simulink model "SingleTrack"  (Simulink 7.5)
settings: Solver=ode45  SolverMode=SingleTasking  StartTime=0.0  StopTime=inf  FixedStep=0.001  RelTol=1e-3
PreLoadFcn:
  | SingleTrack_params
undefined symbols (not defined in the file): Car_Bdy1_mass, Car_Steering_i, Car_Whl_Radius, Car_WhlBaseF, Car_WhlBaseR, mEngineMax, PT_DL_iDiff, PT_GearBox_iForwardGears
libraries: CarMaker4SL x8, simulink x6
(part 2 of 4)

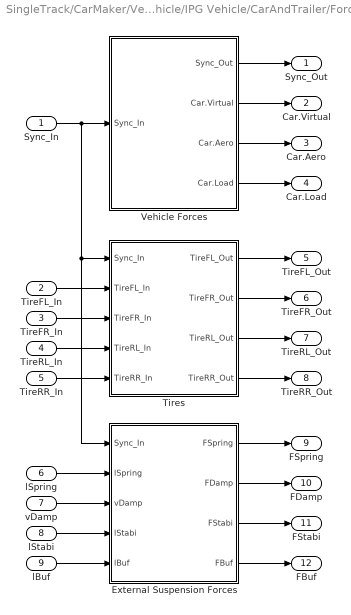
== system SingleTrack/CarMaker/Vehicle/IPG Vehicle/CarAndTrailer/Forces ==
  Sync_In : Inport  OutDataType=sfix(16)  OutScaling=2^0
  TireFL_In : Inport  Port=2  OutDataType=sfix(16)  OutScaling=2^0
  TireFR_In : Inport  Port=3  OutDataType=sfix(16)  OutScaling=2^0
  TireRL_In : Inport  Port=4  OutDataType=sfix(16)  OutScaling=2^0
  TireRR_In : Inport  Port=5  OutDataType=sfix(16)  OutScaling=2^0
  lSpring : Inport  Port=6  OutDataType=sfix(16)  OutScaling=2^0
  vDamp : Inport  Port=7  OutDataType=sfix(16)  OutScaling=2^0
  lStabi : Inport  Port=8  OutDataType=sfix(16)  OutScaling=2^0
  lBuf : Inport  Port=9  OutDataType=sfix(16)  OutScaling=2^0
  External Suspension Forces : Subsystem
  Tires : Subsystem
  Vehicle Forces : Subsystem
  Sync_Out : Outport  OutDataType=sfix(16)  OutScaling=2^0
  Car.Virtual : Outport  Port=2  OutDataType=sfix(16)  OutScaling=2^0
  Car.Aero : Outport  Port=3  OutDataType=sfix(16)  OutScaling=2^0
  Car.Load : Outport  Port=4  OutDataType=sfix(16)  OutScaling=2^0
  TireFL_Out : Outport  Port=5  OutDataType=sfix(16)  OutScaling=2^0
  TireFR_Out : Outport  Port=6  OutDataType=sfix(16)  OutScaling=2^0
  TireRL_Out : Outport  Port=7  OutDataType=sfix(16)  OutScaling=2^0
  TireRR_Out : Outport  Port=8  OutDataType=sfix(16)  OutScaling=2^0
  FSpring : Outport  Port=9  OutDataType=sfix(16)  OutScaling=2^0
  FDamp : Outport  Port=10  OutDataType=sfix(16)  OutScaling=2^0
  FStabi : Outport  Port=11  OutDataType=sfix(16)  OutScaling=2^0
  FBuf : Outport  Port=12  OutDataType=sfix(16)  OutScaling=2^0
  wires:
  External Suspension Forces/1(FSpring) -> FSpring/1
  External Suspension Forces/3(FStabi) -> FStabi/1
  lStabi/1 -> External Suspension Forces/4(lStabi)
  vDamp/1 -> External Suspension Forces/3(vDamp)
  External Suspension Forces/2(FDamp) -> FDamp/1
  lSpring/1 -> External Suspension Forces/2(lSpring)
  Vehicle Forces/4(Car.Load) -> Car.Load/1
  Vehicle Forces/3(Car.Aero) -> Car.Aero/1
  Vehicle Forces/2(Car.Virtual) -> Car.Virtual/1
  TireFL_In/1 -> Tires/2(TireFL_In)
  Vehicle Forces/1(Sync_Out) -> Sync_Out/1
  Sync_In/1 -> Vehicle Forces/1(Sync_In), External Suspension Forces/1(Sync_In), Tires/1(Sync_In)
  TireFR_In/1 -> Tires/3(TireFR_In)
  TireRL_In/1 -> Tires/4(TireRL_In)
  TireRR_In/1 -> Tires/5(TireRR_In)
  Tires/1(TireFL_Out) -> TireFL_Out/1
  Tires/2(TireFR_Out) -> TireFR_Out/1
  Tires/3(TireRL_Out) -> TireRL_Out/1
  Tires/4(TireRR_Out) -> TireRR_Out/1
  lBuf/1 -> External Suspension Forces/5(lBuf)
  External Suspension Forces/4(FBuf) -> FBuf/1

== system SingleTrack/CarMaker/Vehicle/IPG Vehicle/CarAndTrailer/Kinematics ==
  Sync_In : Inport  OutDataType=sfix(16)  OutScaling=2^0
  Steer.IF : Inport  Port=2  OutDataType=sfix(16)  OutScaling=2^0
  Kinematics : S-Function  FunctionName=CM_Sfun  Parameters='Kinematics'  EnableBusSupport=off
  Sync_Out : Outport  OutDataType=sfix(16)  OutScaling=2^0
  TireFL_In : Outport  Port=2  OutDataType=sfix(16)  OutScaling=2^0
  TireFR_In : Outport  Port=3  OutDataType=sfix(16)  OutScaling=2^0
  TireRL_In : Outport  Port=4  OutDataType=sfix(16)  OutScaling=2^0
  TireRR_In : Outport  Port=5  OutDataType=sfix(16)  OutScaling=2^0
  lSpring : Outport  Port=6  OutDataType=sfix(16)  OutScaling=2^0
  vDamp : Outport  Port=7  OutDataType=sfix(16)  OutScaling=2^0
  lStabi : Outport  Port=8  OutDataType=sfix(16)  OutScaling=2^0
  lBuf : Outport  Port=9  OutDataType=sfix(16)  OutScaling=2^0
  wires:
  Steer.IF/1 -> Kinematics/2
  Kinematics/1 -> Sync_Out/1
  Sync_In/1 -> Kinematics/1
  Kinematics/7 -> vDamp/1
  Kinematics/6 -> lSpring/1
  Kinematics/5 -> TireRR_In/1
  Kinematics/4 -> TireRL_In/1
  Kinematics/3 -> TireFR_In/1
  Kinematics/2 -> TireFL_In/1
  Kinematics/8 -> lStabi/1
  Kinematics/9 -> lBuf/1

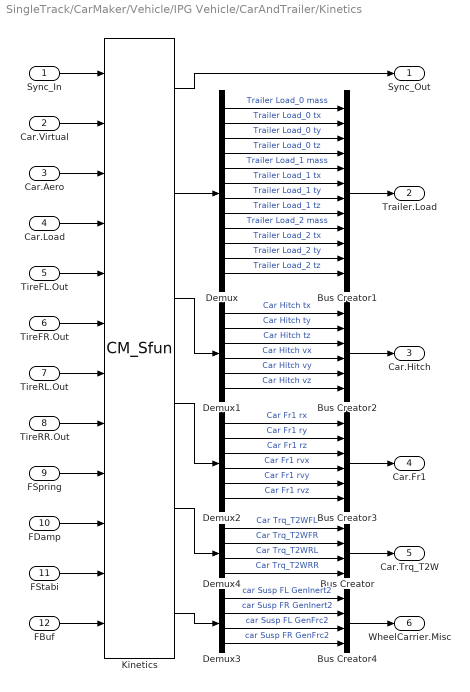
== system SingleTrack/CarMaker/Vehicle/IPG Vehicle/CarAndTrailer/Kinetics ==
  Sync_In : Inport  OutDataType=sfix(16)  OutScaling=2^0
  Car.Virtual : Inport  Port=2  OutDataType=sfix(16)  OutScaling=2^0
  Car.Aero : Inport  Port=3  OutDataType=sfix(16)  OutScaling=2^0
  Car.Load : Inport  Port=4  OutDataType=sfix(16)  OutScaling=2^0
  TireFL.Out : Inport  Port=5  OutDataType=sfix(16)  OutScaling=2^0
  TireFR.Out : Inport  Port=6  OutDataType=sfix(16)  OutScaling=2^0
  TireRL.Out : Inport  Port=7  OutDataType=sfix(16)  OutScaling=2^0
  TireRR.Out : Inport  Port=8  OutDataType=sfix(16)  OutScaling=2^0
  FSpring : Inport  Port=9  OutDataType=sfix(16)  OutScaling=2^0
  FDamp : Inport  Port=10  OutDataType=sfix(16)  OutScaling=2^0
  FStabi : Inport  Port=11  OutDataType=sfix(16)  OutScaling=2^0
  FBuf : Inport  Port=12  OutDataType=sfix(16)  OutScaling=2^0
  Bus Creator : BusCreator
  Bus Creator1 : BusCreator  Inputs=12
  Bus Creator2 : BusCreator  Inputs=6
  Bus Creator3 : BusCreator  Inputs=6
  Bus Creator4 : BusCreator
  Demux : Demux  Outputs=12
  Demux1 : Demux  Outputs=6
  Demux2 : Demux  Outputs=6
  Demux3 : Demux
  Demux4 : Demux
  Kinetics : S-Function  FunctionName=CM_Sfun  Parameters='Kinetics'  EnableBusSupport=off
  Sync_Out : Outport  OutDataType=sfix(16)  OutScaling=2^0
  Trailer.Load : Outport  Port=2  OutDataType=sfix(16)  OutScaling=2^0
  Car.Hitch : Outport  Port=3  OutDataType=sfix(16)  OutScaling=2^0
  Car.Fr1 : Outport  Port=4  OutDataType=sfix(16)  OutScaling=2^0
  Car.Trq_T2W : Outport  Port=5  OutDataType=sfix(16)  OutScaling=2^0
  WheelCarrier.Misc : Outport  Port=6  OutDataType=sfix(16)  OutScaling=2^0
  wires:
  Kinetics/5 -> Demux4/1
  Kinetics/6 -> Demux3/1
  FStabi/1 -> Kinetics/11
  FDamp/1 -> Kinetics/10
  FSpring/1 -> Kinetics/9
  TireRR.Out/1 -> Kinetics/8
  TireRL.Out/1 -> Kinetics/7
  TireFR.Out/1 -> Kinetics/6
  TireFL.Out/1 -> Kinetics/5
  Demux4/1 -> Bus Creator/1  "Car Trq_T2WFL"
  Demux4/2 -> Bus Creator/2  "Car Trq_T2WFR"
  Demux4/3 -> Bus Creator/3  "Car Trq_T2WRL"
  Demux4/4 -> Bus Creator/4  "Car Trq_T2WRR"
  Bus Creator/1 -> Car.Trq_T2W/1
  Bus Creator4/1 -> WheelCarrier.Misc/1
  Demux3/4 -> Bus Creator4/4  "car Susp FR GenFrc2"
  Demux3/3 -> Bus Creator4/3  "car Susp FL GenFrc2"
  Demux3/2 -> Bus Creator4/2  "car Susp FR GenInert2"
  Demux3/1 -> Bus Creator4/1  "car Susp FL GenInert2"
  Car.Load/1 -> Kinetics/4
  Kinetics/4 -> Demux2/1
  Bus Creator3/1 -> Car.Fr1/1
  Demux2/6 -> Bus Creator3/6  "Car Fr1 rvz"
  Demux2/5 -> Bus Creator3/5  "Car Fr1 rvy"
  Demux2/4 -> Bus Creator3/4  "Car Fr1 rvx"
  Demux2/3 -> Bus Creator3/3  "Car Fr1 rz"
  Demux2/2 -> Bus Creator3/2  "Car Fr1 ry"
  Demux2/1 -> Bus Creator3/1  "Car Fr1 rx"
  Bus Creator2/1 -> Car.Hitch/1
  Kinetics/3 -> Demux1/1
  Demux1/6 -> Bus Creator2/6  "Car Hitch vz"
  Demux1/5 -> Bus Creator2/5  "Car Hitch vy"
  Demux1/4 -> Bus Creator2/4  "Car Hitch vx"
  Demux1/3 -> Bus Creator2/3  "Car Hitch tz"
  Demux1/2 -> Bus Creator2/2  "Car Hitch ty"
  Demux1/1 -> Bus Creator2/1  "Car Hitch tx"
  Demux/12 -> Bus Creator1/12  "Trailer Load_2 tz"
  Demux/11 -> Bus Creator1/11  "Trailer Load_2 ty"
  Demux/10 -> Bus Creator1/10  "Trailer Load_2 tx"
  Demux/9 -> Bus Creator1/9  "Trailer Load_2 mass"
  Demux/8 -> Bus Creator1/8  "Trailer Load_1 tz"
  Demux/7 -> Bus Creator1/7  "Trailer Load_1 ty"
  Demux/6 -> Bus Creator1/6  "Trailer Load_1 tx"
  Demux/5 -> Bus Creator1/5  "Trailer Load_1 mass"
  Kinetics/2 -> Demux/1
  Demux/4 -> Bus Creator1/4  "Trailer Load_0 tz"
  Demux/3 -> Bus Creator1/3  "Trailer Load_0 ty"
  Demux/2 -> Bus Creator1/2  "Trailer Load_0 tx"
  Demux/1 -> Bus Creator1/1  "Trailer Load_0 mass"
  Bus Creator1/1 -> Trailer.Load/1
  Car.Virtual/1 -> Kinetics/2
  Car.Aero/1 -> Kinetics/3
  Kinetics/1 -> Sync_Out/1
  Sync_In/1 -> Kinetics/1
  FBuf/1 -> Kinetics/12

== system SingleTrack/CarMaker/Vehicle/IPG Vehicle/CarAndTrailer/Steering ==
  note: When replacing the entire steering system,
      | be sure to add '-disablesteering' to the command line arguments
      | in the CarMaker Model Configuration block.
  Sync_In : Inport  OutDataType=sfix(16)  OutScaling=2^0
  VhclCtrl.Steering : Inport  Port=2  OutDataType=sfix(16)  OutScaling=2^0
  Bus Creator1 : BusCreator  Inputs=16
  Bus Creator2 : BusCreator
  Demux : Demux  Outputs=20
  Steering : S-Function  FunctionName=CM_Sfun  Parameters='Steering'  EnableBusSupport=off
  Terminator : Terminator
  Sync_Out : Outport  OutDataType=sfix(16)  OutScaling=2^0
  Steer.IF : Outport  Port=2  OutDataType=sfix(16)  OutScaling=2^0
  wires:
  Demux/5 -> Bus Creator1/5  "Steering IF TrqStatic"
  Demux/4 -> Bus Creator1/4  "Steering IF Trq"
  Demux/3 -> Bus Creator1/3  "Steering IF AngAcc"
  Demux/2 -> Bus Creator1/2  "Steering IF AngVel"
  Demux/1 -> Bus Creator1/1  "Steering IF Ang"
  Sync_In/1 -> Steering/1
  Steering/1 -> Sync_Out/1
  VhclCtrl.Steering/1 -> Steering/2
  Demux/15 -> Bus Creator1/15  "Steering IF R qpp"
  Demux/14 -> Bus Creator1/14  "Steering IF R qp"
  Demux/13 -> Bus Creator1/13  "Steering IF R q"
  Demux/12 -> Bus Creator1/12  "Steering IF L iSteer2q"
  Demux/11 -> Bus Creator1/11  "Steering IF L qpp"
  Demux/10 -> Bus Creator1/10  "Steering IF L qp"
  Demux/9 -> Bus Creator1/9  "Steering IF L q"
  Demux/16 -> Bus Creator1/16  "Steering IF R iSteer2q"
  Bus Creator2/1 -> Terminator/1  "Steer IF (in)"
  Demux/19 -> Bus Creator2/3  "Steering IF R Frc"
  Demux/18 -> Bus Creator2/2  "Steering IF L Inert"
  Demux/17 -> Bus Creator2/1  "Steering IF L Frc"
  Demux/20 -> Bus Creator2/4  "Steering IF R Inert"
  Demux/6 -> Bus Creator1/6  "Steering IF AssistFrc"
  Demux/7 -> Bus Creator1/7  "Steering IF AssistTrqCol"
  Demux/8 -> Bus Creator1/8  "Steering IF AssistTrqPin"
  Steering/2 -> Demux/1
  Bus Creator1/1 -> Steer.IF/1

== system SingleTrack/CarMaker/Vehicle/IPG Vehicle/CarAndTrailer/Trailer ==
  Sync_In : Inport  OutDataType=sfix(16)  OutScaling=2^0
  Trailer.Load : Inport  Port=2  OutDataType=sfix(16)  OutScaling=2^0
  Car.Hitch : Inport  Port=3  OutDataType=sfix(16)  OutScaling=2^0
  Car.Fr1 : Inport  Port=4  OutDataType=sfix(16)  OutScaling=2^0
  Car.Trq_T2W : Inport  Port=5  OutDataType=sfix(16)  OutScaling=2^0
  WheelCarrier.Misc : Inport  Port=6  OutDataType=sfix(16)  OutScaling=2^0
  CreateBus Car.Hitch.FrcTrq : Subsystem
  CreateBus Vhcl.Motion : Subsystem
  CreateBus Vhcl.PoI : Subsystem
  CreateBus Vhcl.Steering : Subsystem
  CreateBus Vhcl.Wheel.FL : Subsystem
  CreateBus Vhcl.Wheel.FR : Subsystem
  CreateBus Vhcl.Wheel.RL : Subsystem
  CreateBus Vhcl.Wheel.RR : Subsystem
  Trailer : S-Function  FunctionName=CM_Sfun  Parameters='Trailer'  EnableBusSupport=off
  Sync_Out : Outport  OutDataType=sfix(16)  OutScaling=2^0
  Vhcl.Steering : Outport  Port=2  OutDataType=sfix(16)  OutScaling=2^0
  Vhcl.Motion : Outport  Port=3  OutDataType=sfix(16)  OutScaling=2^0
  Vhcl.PoI : Outport  Port=4  OutDataType=sfix(16)  OutScaling=2^0
  Vhcl.Wheel.FL : Outport  Port=5  OutDataType=sfix(16)  OutScaling=2^0
  Vhcl.Wheel.FR : Outport  Port=6  OutDataType=sfix(16)  OutScaling=2^0
  Vhcl.Wheel.RL : Outport  Port=7  OutDataType=sfix(16)  OutScaling=2^0
  Vhcl.Wheel.RR : Outport  Port=8  OutDataType=sfix(16)  OutScaling=2^0
  Car.Hitch.FrcTrq : Outport  Port=9  OutDataType=sfix(16)  OutScaling=2^0
  wires:
  Sync_In/1 -> Trailer/1
  Trailer/1 -> Sync_Out/1
  Trailer.Load/1 -> Trailer/2
  Car.Hitch/1 -> Trailer/3
  Car.Fr1/1 -> Trailer/4
  CreateBus Car.Hitch.FrcTrq/1(Car.Hitch.FrcTrq) -> Car.Hitch.FrcTrq/1
  WheelCarrier.Misc/1 -> Trailer/6
  Car.Trq_T2W/1 -> Trailer/5
  CreateBus Vhcl.Motion/1(Out1) -> Vhcl.Motion/1
  CreateBus Vhcl.PoI/1(Out1) -> Vhcl.PoI/1
  CreateBus Vhcl.Wheel.FL/1(Out1) -> Vhcl.Wheel.FL/1  "Vhcl.Wheel.FL"
  CreateBus Vhcl.Wheel.FR/1(Out1) -> Vhcl.Wheel.FR/1  "Vhcl.Wheel.FR"
  CreateBus Vhcl.Wheel.RL/1(Out1) -> Vhcl.Wheel.RL/1  "Vhcl.Wheel.RL"
  CreateBus Vhcl.Wheel.RR/1(Out1) -> Vhcl.Wheel.RR/1  "Vhcl.Wheel.RR"
  Trailer/8 -> CreateBus Vhcl.Wheel.RR/1(In1)
  Trailer/9 -> CreateBus Car.Hitch.FrcTrq/1(In1)
  Trailer/7 -> CreateBus Vhcl.Wheel.RL/1(In1)
  Trailer/6 -> CreateBus Vhcl.Wheel.FR/1(In1)
  Trailer/5 -> CreateBus Vhcl.Wheel.FL/1(In1)
  Trailer/4 -> CreateBus Vhcl.PoI/1(In1)
  Trailer/3 -> CreateBus Vhcl.Motion/1(In1)
  CreateBus Vhcl.Steering/1(Out1) -> Vhcl.Steering/1
  Trailer/2 -> CreateBus Vhcl.Steering/1(In1)

== system SingleTrack/CarMaker/Vehicle/User Vehicle (CM4SL)/Brake/CreateBus Vhcl.Wheel.PT ==
  In : Inport
  BusCreator : BusCreator  Inputs=16
  Demux : Demux  Outputs=16
  Out : Outport
  wires:
  In/1 -> Demux/1
  BusCreator/1 -> Out/1
  Demux/1 -> BusCreator/1  "Vhcl Wheel FL Trq_Brake"
  Demux/2 -> BusCreator/2  "Vhcl Wheel FL Trq_BrakeReg_trg"
  Demux/3 -> BusCreator/3  "Vhcl Wheel FL Trq_T2W"
  Demux/4 -> BusCreator/4  "Vhcl Wheel FL WhlBearing"
  Demux/5 -> BusCreator/5  "Vhcl Wheel FR Trq_Brake"
  Demux/6 -> BusCreator/6  "Vhcl Wheel FR Trq_BrakeReg_trg"
  Demux/7 -> BusCreator/7  "Vhcl Wheel FR Trq_T2W"
  Demux/8 -> BusCreator/8  "Vhcl Wheel FR WhlBearing"
  Demux/9 -> BusCreator/9  "Vhcl Wheel RL Trq_Brake"
  Demux/10 -> BusCreator/10  "Vhcl Wheel RL Trq_BrakeReg_trg"
  Demux/11 -> BusCreator/11  "Vhcl Wheel RL Trq_T2W"
  Demux/12 -> BusCreator/12  "Vhcl Wheel RL WhlBearing"
  Demux/13 -> BusCreator/13  "Vhcl Wheel RR Trq_Brake"
  Demux/14 -> BusCreator/14  "Vhcl Wheel RR Trq_BrakeReg_trg"
  Demux/15 -> BusCreator/15  "Vhcl Wheel RR Trq_T2W"
  Demux/16 -> BusCreator/16  "Vhcl Wheel RR WhlBearing"

== system SingleTrack/CarMaker/Vehicle/User Vehicle (CM4SL)/CarAndTrailer/CarAndTrailerUpd1 ==
  Sync_In : Inport  OutDataType=sfix(16)  OutScaling=2^0
  Vhcl.Steering : Inport  Port=2  OutDataType=sfix(16)  OutScaling=2^0
  Vhcl.Motion : Inport  Port=3  OutDataType=sfix(16)  OutScaling=2^0
  Vhcl.PoI : Inport  Port=4  OutDataType=sfix(16)  OutScaling=2^0
  Vhcl.Wheel.FL : Inport  Port=5  OutDataType=sfix(16)  OutScaling=2^0
  Vhcl.Wheel.FR : Inport  Port=6  OutDataType=sfix(16)  OutScaling=2^0
  Vhcl.Wheel.RL : Inport  Port=7  OutDataType=sfix(16)  OutScaling=2^0
  Vhcl.Wheel.RR : Inport  Port=8  OutDataType=sfix(16)  OutScaling=2^0
  Car.Hitch.FrcTrq : Inport  Port=9  OutDataType=sfix(16)  OutScaling=2^0
  Vhcl.Fr1A : Inport  Port=10  OutDataType=sfix(16)  OutScaling=2^0
  CarAndTrailerUpd : S-Function  FunctionName=CM_Sfun  Parameters='CarAndTrUpd'  EnableBusSupport=off
  CreateBus Brake.IF.In : Subsystem
  Sync_Out : Outport  OutDataType=sfix(16)  OutScaling=2^0
  Brake.IF.In : Outport  Port=2  OutDataType=sfix(16)  OutScaling=2^0
  wires:
  Sync_In/1 -> CarAndTrailerUpd/1
  CarAndTrailerUpd/1 -> Sync_Out/1
  CreateBus Brake.IF.In/1(Out) -> Brake.IF.In/1
  CarAndTrailerUpd/2 -> CreateBus Brake.IF.In/1(In)
  Vhcl.Wheel.RL/1 -> CarAndTrailerUpd/7
  Vhcl.Wheel.RR/1 -> CarAndTrailerUpd/8
  Car.Hitch.FrcTrq/1 -> CarAndTrailerUpd/9
  Vhcl.Wheel.FR/1 -> CarAndTrailerUpd/6
  Vhcl.Wheel.FL/1 -> CarAndTrailerUpd/5
  Vhcl.PoI/1 -> CarAndTrailerUpd/4
  Vhcl.Motion/1 -> CarAndTrailerUpd/3
  Vhcl.Steering/1 -> CarAndTrailerUpd/2
  Vhcl.Fr1A/1 -> CarAndTrailerUpd/10  "user vehicle only"

== system SingleTrack/CarMaker/Vehicle/User Vehicle (CM4SL)/CarAndTrailer/CreateBus Car.Hitch.FrcTrq ==
  Bus Creator : BusCreator  Inputs=6
  Constant{1..2,7..10} (6 alike) : Constant  Value=0  OutDataType=sfix(16)  OutScaling=2^0
  Demux7 : Demux  Outputs=6
  Mux1 : Mux  Inputs=6
  Car.Hitch.FrcTrq : Outport  OutDataType=sfix(16)  OutScaling=2^0
  wires:
  Demux7/1 -> Bus Creator/1  "Car Hitch Frc2Car x"
  Demux7/2 -> Bus Creator/2  "Car Hitch Frc2Car y"
  Demux7/3 -> Bus Creator/3  "Car Hitch Frc2Car z"
  Demux7/4 -> Bus Creator/4  "Car Hitch Trq2Car x"
  Demux7/5 -> Bus Creator/5  "Car Hitch Trq2Car y"
  Demux7/6 -> Bus Creator/6  "Car Hitch Trq2Car z"
  Bus Creator/1 -> Car.Hitch.FrcTrq/1
  Mux1/1 -> Demux7/1
  Constant8/1 -> Mux1/2
  Constant9/1 -> Mux1/3
  Constant10/1 -> Mux1/4
  Constant7/1 -> Mux1/1
  Constant2/1 -> Mux1/5
  Constant1/1 -> Mux1/6

== system SingleTrack/CarMaker/Vehicle/User Vehicle (CM4SL)/CarAndTrailer/CreateBus Vhcl.Fr1 ==
  Vhcl.Fr1_In : Inport  OutDataType=sfix(16)  OutScaling=2^0
  BdyFrame2Vhcl.Fr1A : Subsystem
  Ground : Ground
  Ground1 : Ground
  Tr2Fr0 : Subsystem
  a_0 : Subsystem
  t_0 : Subsystem
  v_0 : Subsystem
  Vhcl.Fr1A : Outport  OutDataType=sfix(16)  OutScaling=2^0
  wires:
  BdyFrame2Vhcl.Fr1A/1(Vhcl.Fr1) -> Vhcl.Fr1A/1
  Vhcl.Fr1_In/1 -> a_0/1(Car), v_0/1(Car), t_0/1(Car), Tr2Fr0/1(Car)
  Tr2Fr0/1(Tr2Fr0) -> v_0/2(Tr2Fr0), a_0/2(Tr2Fr0), BdyFrame2Vhcl.Fr1A/6(Tr2Fr0)
  t_0/1(t_0) -> BdyFrame2Vhcl.Fr1A/1(t_0)
  v_0/1(v_0) -> BdyFrame2Vhcl.Fr1A/2(v_0)
  a_0/1(a_0) -> BdyFrame2Vhcl.Fr1A/3(a_0)
  Ground1/1 -> BdyFrame2Vhcl.Fr1A/4(omega_0)
  Ground/1 -> BdyFrame2Vhcl.Fr1A/5(alpha_0)

== system SingleTrack/CarMaker/Vehicle/User Vehicle (CM4SL)/CarAndTrailer/CreateBus Vhcl.Motion ==
  Vhcl_Motion_In : Inport  OutDataType=sfix(16)  OutScaling=2^0
  Bus Creator : BusCreator  Inputs=16
  Bus Selector1 : BusSelector  OutputSignals=Car_vx_1,Car_Dist,Car_sRoad,Road_Fr1_rx,Road_Fr1_ry,Car_Yaw,Car_Yawp,Car_Yawpp
  Constant{1,5,8,11..14} (7 alike) : Constant  Value=0  OutDataType=sfix(16)  OutScaling=2^0
  Demux1 : Demux  Outputs=16
  Mux3 : Mux  Inputs=16
  Vhcl .Motion : Outport  OutDataType=sfix(16)  OutScaling=2^0
  wires:
  Vhcl_Motion_In/1 -> Bus Selector1/1
  Mux3/1 -> Demux1/1
  Bus Creator/1 -> Vhcl .Motion/1
  Demux1/16 -> Bus Creator/16  "Vhcl YawAcc"
  Demux1/15 -> Bus Creator/15  "Vhcl YawRate"
  Demux1/14 -> Bus Creator/14  "Vhcl Yaw"
  Demux1/13 -> Bus Creator/13  "Vhcl PitchAcc"
  Demux1/12 -> Bus Creator/12  "Vhcl PitchVel"
  Demux1/11 -> Bus Creator/11  "Vhcl Pitch"
  Demux1/10 -> Bus Creator/10  "Vhcl RollAcc"
  Demux1/9 -> Bus Creator/9  "Vhcl RollVel"
  Demux1/8 -> Bus Creator/8  "Vhcl Roll"
  Demux1/7 -> Bus Creator/7  "Vhcl Hitch_Pos z"
  Demux1/6 -> Bus Creator/6  "Vhcl Hitch_Pos y"
  Demux1/5 -> Bus Creator/5  "Vhcl Hitch_Pos x"
  Demux1/4 -> Bus Creator/4  "Vhcl sRoadAero"
  Demux1/3 -> Bus Creator/3  "Vhcl sRoad"
  Demux1/2 -> Bus Creator/2  "Vhcl Distance"
  Demux1/1 -> Bus Creator/1  "Vhcl v"
  Bus Selector1/3 -> Mux3/4, Mux3/3  "<Car_sRoad>"
  Bus Selector1/5 -> Mux3/11  "<Road_Fr1_ry>"
  Bus Selector1/4 -> Mux3/8  "<Road_Fr1_rx>"
  Bus Selector1/8 -> Mux3/16  "<Car_Yawpp>"
  Bus Selector1/7 -> Mux3/15  "<Car_Yawp>"
  Bus Selector1/6 -> Mux3/14  "<Car_Yaw>"
  Constant1/1 -> Mux3/13
  Constant14/1 -> Mux3/12
  Constant13/1 -> Mux3/10
  Constant12/1 -> Mux3/9
  Constant11/1 -> Mux3/7
  Constant8/1 -> Mux3/6
  Constant5/1 -> Mux3/5
  Bus Selector1/2 -> Mux3/2  "<Car_Dist>"
  Bus Selector1/1 -> Mux3/1  "<Car_vx_1>"

== system SingleTrack/CarMaker/Vehicle/User Vehicle (CM4SL)/CarAndTrailer/CreateBus Vhcl.PoI ==
  Vhcl_POI_In : Inport  OutDataType=sfix(16)  OutScaling=2^0
  Bus Creator : BusCreator  Inputs=18
  Bus Selector : BusSelector  OutputSignals=Car_x,Car_y,Road_Fr1_z,Car_vx,Car_vy,Car_ax,Car_ay,Car_vx_1,Car_ax_1,Car_ay_1
  Constant{11..13,15..19} (8 alike) : Constant  Value=0  OutDataType=sfix(16)  OutScaling=2^0
  Demux3 : Demux  Outputs=18
  Mux1 : Mux  Inputs=18
  Vhcl.PoI : Outport  OutDataType=sfix(16)  OutScaling=2^0
  wires:
  Demux3/1 -> Bus Creator/1  "Vhcl PoI_Pos x"
  Bus Creator/1 -> Vhcl.PoI/1
  Demux3/2 -> Bus Creator/2  "Vhcl PoI_Pos y"
  Demux3/3 -> Bus Creator/3  "Vhcl PoI_Pos z"
  Demux3/4 -> Bus Creator/4  "Vhcl PoI_Vel x"
  Demux3/5 -> Bus Creator/5  "Vhcl PoI_Vel y"
  Demux3/6 -> Bus Creator/6  "Vhcl PoI_Vel z"
  Demux3/7 -> Bus Creator/7  "Vhcl PoI_Acc x"
  Demux3/8 -> Bus Creator/8  "Vhcl PoI_Acc y"
  Demux3/9 -> Bus Creator/9  "Vhcl PoI_Acc z"
  Demux3/10 -> Bus Creator/10  "Vhcl PoI_Vel_1 x"
  Demux3/11 -> Bus Creator/11  "Vhcl PoI_Vel_1 y"
  Demux3/12 -> Bus Creator/12  "Vhcl PoI_Vel_1 z"
  Demux3/13 -> Bus Creator/13  "Vhcl PoI_Acc_1 x"
  Demux3/14 -> Bus Creator/14  "Vhcl PoI_Acc_1 y"
  Demux3/15 -> Bus Creator/15  "Vhcl PoI_Acc_1 z"
  Demux3/16 -> Bus Creator/16  "Vhcl PoI_GCS Long"
  Demux3/17 -> Bus Creator/17  "Vhcl PoI_GCS Lat"
  Demux3/18 -> Bus Creator/18  "Vhcl PoI_GCS Elev"
  Mux1/1 -> Demux3/1
  Vhcl_POI_In/1 -> Bus Selector/1
  Constant12/1 -> Mux1/16
  Constant13/1 -> Mux1/17
  Constant11/1 -> Mux1/18
  Bus Selector/1 -> Mux1/1  "<Car_x>"
  Bus Selector/2 -> Mux1/2  "<Car_y>"
  Bus Selector/3 -> Mux1/3  "<Road_Fr1_z>"
  Bus Selector/4 -> Mux1/4  "<Car_vx>"
  Bus Selector/5 -> Mux1/5  "<Car_vy>"
  Constant15/1 -> Mux1/6
  Bus Selector/6 -> Mux1/7  "<Car_ax>"
  Constant16/1 -> Mux1/9
  Constant17/1 -> Mux1/11
  Constant18/1 -> Mux1/12
  Bus Selector/9 -> Mux1/13  "<Car_ax_1>"
  Bus Selector/10 -> Mux1/14  "<Car_ay_1>"
  Constant19/1 -> Mux1/15
  Bus Selector/7 -> Mux1/8  "<Car_ay>"
  Bus Selector/8 -> Mux1/10  "<Car_vx_1>"

== system SingleTrack/CarMaker/Vehicle/User Vehicle (CM4SL)/CarAndTrailer/CreateBus Vhcl.Steering ==
  Vhcl_Steering_In : Inport  OutDataType=sfix(16)  OutScaling=2^0
  Bus Creator : BusCreator
  Bus Selector : BusSelector  OutputSignals=VhclCtrl Steering Ang,VhclCtrl Steering AngVel,VhclCtrl Steering AngAcc,VhclCtrl Steering Trq
  Demux : Demux
  Mux1 : Mux
  Vhcl.Steering : Outport  OutDataType=sfix(16)  OutScaling=2^0
  wires:
  Demux/4 -> Bus Creator/4  "Vhcl Steering Trq"
  Demux/2 -> Bus Creator/2  "Vhcl Steering AngVel"
  Demux/3 -> Bus Creator/3  "Vhcl Steering AngAcc"
  Demux/1 -> Bus Creator/1  "Vhcl Steering Ang"
  Bus Creator/1 -> Vhcl.Steering/1
  Vhcl_Steering_In/1 -> Bus Selector/1
  Bus Selector/1 -> Mux1/1  "<VhclCtrl Steering Ang>"
  Bus Selector/2 -> Mux1/2  "<VhclCtrl Steering AngVel>"
  Bus Selector/3 -> Mux1/3  "<VhclCtrl Steering AngAcc>"
  Bus Selector/4 -> Mux1/4  "<VhclCtrl Steering Trq>"
  Mux1/1 -> Demux/1

== system SingleTrack/CarMaker/Vehicle/User Vehicle (CM4SL)/CarAndTrailer/CreateBus Vhcl.Wheel.FL ==
  Vhcl.Wheel.FL_In : Inport  OutDataType=sfix(16)  OutScaling=2^0
  Bus Creator : BusCreator  Inputs=14
  Bus Selector : BusSelector  OutputSignals=Car_Whl_F_rz,Car_Whl_Fz,Car_Whl_F_SideSlip
  Constant{1..6,8..12} (11 alike) : Constant  Value=0  OutDataType=sfix(16)  OutScaling=2^0
  Demux3 : Demux  Outputs=14
  Mux1 : Mux  Inputs=14
  Vhcl.Wheel.FL : Outport  OutDataType=sfix(16)  OutScaling=2^0
  wires:
  Demux3/1 -> Bus Creator/1  "Vhcl Wheel FL t x"
  Bus Creator/1 -> Vhcl.Wheel.FL/1
  Mux1/1 -> Demux3/1
  Demux3/2 -> Bus Creator/2  "Vhcl Wheel FL t y"
  Demux3/3 -> Bus Creator/3  "Vhcl Wheel FL t z"
  Demux3/4 -> Bus Creator/4  "Vhcl Wheel FL r_zxy x"
  Demux3/5 -> Bus Creator/5  "Vhcl Wheel FL r_zxy y"
  Demux3/6 -> Bus Creator/6  "Vhcl Wheel FL r_zxy z"
  Demux3/7 -> Bus Creator/7  "Vhcl Wheel FL Fx"
  Demux3/8 -> Bus Creator/8  "Vhcl Wheel FL Fy"
  Demux3/9 -> Bus Creator/9  "Vhcl Wheel FL Fz"
  Demux3/10 -> Bus Creator/10  "Vhcl Wheel FL vBelt"
  Demux3/11 -> Bus Creator/11  "Vhcl Wheel FL LongSlip"
  Demux3/12 -> Bus Creator/12  "Vhcl Wheel FL SideSlip"
  Demux3/13 -> Bus Creator/13  "Vhcl Wheel FL Trq_T2W"
  Demux3/14 -> Bus Creator/14  "Vhcl Wheel FL Trq_WhlBearing"
  Vhcl.Wheel.FL_In/1 -> Bus Selector/1
  Bus Selector/1 -> Mux1/6  "<Car_Whl_F_rz>"
  Constant1/1 -> Mux1/1
  Constant2/1 -> Mux1/2
  Constant3/1 -> Mux1/3
  Constant4/1 -> Mux1/4
  Constant5/1 -> Mux1/5
  Constant6/1 -> Mux1/7
  Constant8/1 -> Mux1/8
  Bus Selector/3 -> Mux1/12  "<Car_Whl_F_SideSlip>"
  Constant9/1 -> Mux1/10
  Constant10/1 -> Mux1/11
  Constant12/1 -> Mux1/13
  Constant11/1 -> Mux1/14
  Bus Selector/2 -> Mux1/9  "<Car_Whl_Fz>"

== system SingleTrack/CarMaker/Vehicle/User Vehicle (CM4SL)/CarAndTrailer/CreateBus Vhcl.Wheel.FR ==
  Vhcl.Wheel.FR_In : Inport  OutDataType=sfix(16)  OutScaling=2^0
  Bus Creator : BusCreator  Inputs=14
  Bus Selector : BusSelector  OutputSignals=Car_Whl_F_rz,Car_Whl_Fz,Car_Whl_F_SideSlip
  Constant{1..7,9..12} (11 alike) : Constant  Value=0  OutDataType=sfix(16)  OutScaling=2^0
  Demux3 : Demux  Outputs=14
  Mux1 : Mux  Inputs=14
  Vhcl.Wheel.FR : Outport  OutDataType=sfix(16)  OutScaling=2^0
  wires:
  Demux3/1 -> Bus Creator/1  "Vhcl Wheel FR t x"
  Bus Creator/1 -> Vhcl.Wheel.FR/1
  Demux3/2 -> Bus Creator/2  "Vhcl Wheel FR t y"
  Demux3/3 -> Bus Creator/3  "Vhcl Wheel FR t z"
  Demux3/4 -> Bus Creator/4  "Vhcl Wheel FR r_zxy x"
  Demux3/5 -> Bus Creator/5  "Vhcl Wheel FR r_zxy y"
  Demux3/6 -> Bus Creator/6  "Vhcl Wheel FR r_zxy z"
  Demux3/7 -> Bus Creator/7  "Vhcl Wheel FR Fx"
  Demux3/8 -> Bus Creator/8  "Vhcl Wheel FR Fy"
  Demux3/9 -> Bus Creator/9  "Vhcl Wheel FR Fz"
  Demux3/10 -> Bus Creator/10  "Vhcl Wheel FR vBelt"
  Demux3/11 -> Bus Creator/11  "Vhcl Wheel FR LongSlip"
  Demux3/12 -> Bus Creator/12  "Vhcl Wheel FR SideSlip"
  Demux3/13 -> Bus Creator/13  "Vhcl Wheel FR Trq_T2W"
  Demux3/14 -> Bus Creator/14  "Vhcl Wheel FR Trq_WhlBearing"
  Mux1/1 -> Demux3/1
  Vhcl.Wheel.FR_In/1 -> Bus Selector/1
  Bus Selector/1 -> Mux1/6  "<Car_Whl_F_rz>"
  Constant1/1 -> Mux1/1
  Constant2/1 -> Mux1/2
  Constant3/1 -> Mux1/3
  Constant4/1 -> Mux1/4
  Constant5/1 -> Mux1/5
  Constant6/1 -> Mux1/7
  Constant7/1 -> Mux1/8
  Bus Selector/2 -> Mux1/9  "<Car_Whl_Fz>"
  Bus Selector/3 -> Mux1/12  "<Car_Whl_F_SideSlip>"
  Constant9/1 -> Mux1/10
  Constant10/1 -> Mux1/11
  Constant12/1 -> Mux1/13
  Constant11/1 -> Mux1/14

== system SingleTrack/CarMaker/Vehicle/User Vehicle (CM4SL)/CarAndTrailer/CreateBus Vhcl.Wheel.RL ==
  Vhcl.Wheel.RL_In : Inport  OutDataType=sfix(16)  OutScaling=2^0
  Bus Creator : BusCreator  Inputs=14
  Bus Selector : BusSelector  OutputSignals=Car_Whl_Fz,Car_Whl_R_SideSlip
  Constant{1..7,9..13} (12 alike) : Constant  Value=0  OutDataType=sfix(16)  OutScaling=2^0
  Demux3 : Demux  Outputs=14
  Mux1 : Mux  Inputs=14
  Vhcl.Wheel.RL : Outport  OutDataType=sfix(16)  OutScaling=2^0
  wires:
  Demux3/1 -> Bus Creator/1  "Vhcl Wheel RL t x"
  Bus Creator/1 -> Vhcl.Wheel.RL/1
  Demux3/2 -> Bus Creator/2  "Vhcl Wheel RL t y"
  Demux3/3 -> Bus Creator/3  "Vhcl Wheel RL t z"
  Demux3/4 -> Bus Creator/4  "Vhcl Wheel RL r_zxy x"
  Demux3/5 -> Bus Creator/5  "Vhcl Wheel RL r_zxy y"
  Demux3/6 -> Bus Creator/6  "Vhcl Wheel RL r_zxy z"
  Demux3/7 -> Bus Creator/7  "Vhcl Wheel RL Fx"
  Demux3/8 -> Bus Creator/8  "Vhcl Wheel RL Fy"
  Demux3/9 -> Bus Creator/9  "Vhcl Wheel RL Fz"
  Demux3/10 -> Bus Creator/10  "Vhcl Wheel RL vBelt"
  Demux3/11 -> Bus Creator/11  "Vhcl Wheel RL LongSlip"
  Demux3/12 -> Bus Creator/12  "Vhcl Wheel RL SideSlip"
  Demux3/13 -> Bus Creator/13  "Vhcl Wheel RL Trq_T2W"
  Demux3/14 -> Bus Creator/14  "Vhcl Wheel RL Trq_WhlBearing"
  Mux1/1 -> Demux3/1
  Vhcl.Wheel.RL_In/1 -> Bus Selector/1
  Constant1/1 -> Mux1/1
  Constant2/1 -> Mux1/2
  Constant3/1 -> Mux1/3
  Constant4/1 -> Mux1/4
  Constant5/1 -> Mux1/5
  Constant6/1 -> Mux1/7
  Constant7/1 -> Mux1/8
  Bus Selector/1 -> Mux1/9  "<Car_Whl_Fz>"
  Constant9/1 -> Mux1/10
  Constant10/1 -> Mux1/11
  Constant12/1 -> Mux1/13
  Constant11/1 -> Mux1/14
  Constant13/1 -> Mux1/6
  Bus Selector/2 -> Mux1/12  "<Car_Whl_R_SideSlip>"

== system SingleTrack/CarMaker/Vehicle/User Vehicle (CM4SL)/CarAndTrailer/CreateBus Vhcl.Wheel.RR ==
  Vhcl.Wheel.RR_In : Inport  OutDataType=sfix(16)  OutScaling=2^0
  Bus Selector : BusSelector  OutputSignals=Car_Whl_Fz,Car_Whl_R_SideSlip
  Constant{1..7,9..13} (12 alike) : Constant  Value=0  OutDataType=sfix(16)  OutScaling=2^0
  Demux3 : Demux  Outputs=14
  Mux : Mux  Inputs=14
  Mux1 : Mux  Inputs=14
  Vhcl.Wheel.RR : Outport  OutDataType=sfix(16)  OutScaling=2^0
  wires:
  Demux3/1 -> Mux/1  "Vhcl Wheel RR t x"
  Mux/1 -> Vhcl.Wheel.RR/1
  Demux3/2 -> Mux/2  "Vhcl Wheel RR t y"
  Demux3/3 -> Mux/3  "Vhcl Wheel RR t z"
  Demux3/4 -> Mux/4  "Vhcl Wheel RR r_zxy x"
  Demux3/5 -> Mux/5  "Vhcl Wheel RR r_zxy y"
  Demux3/6 -> Mux/6  "Vhcl Wheel RR r_zxy z"
  Demux3/7 -> Mux/7  "Vhcl Wheel RR Fx"
  Demux3/8 -> Mux/8  "Vhcl Wheel RR Fy"
  Demux3/9 -> Mux/9  "Vhcl Wheel RR Fz"
  Demux3/10 -> Mux/10  "Vhcl Wheel RR vBelt"
  Demux3/11 -> Mux/11  "Vhcl Wheel RR LongSlip"
  Demux3/12 -> Mux/12  "Vhcl Wheel RR SideSlip"
  Demux3/13 -> Mux/13  "Vhcl Wheel RR Trq_T2W"
  Demux3/14 -> Mux/14  "Vhcl Wheel RR Trq_WhlBearing"
  Mux1/1 -> Demux3/1
  Vhcl.Wheel.RR_In/1 -> Bus Selector/1
  Constant1/1 -> Mux1/1
  Constant2/1 -> Mux1/2
  Constant3/1 -> Mux1/3
  Constant4/1 -> Mux1/4
  Constant5/1 -> Mux1/5
  Constant6/1 -> Mux1/7
  Constant7/1 -> Mux1/8
  Bus Selector/1 -> Mux1/9  "<Car_Whl_Fz>"
  Constant9/1 -> Mux1/10
  Constant10/1 -> Mux1/11
  Constant12/1 -> Mux1/13
  Constant11/1 -> Mux1/14
  Constant13/1 -> Mux1/6
  Bus Selector/2 -> Mux1/12  "<Car_Whl_R_SideSlip>"

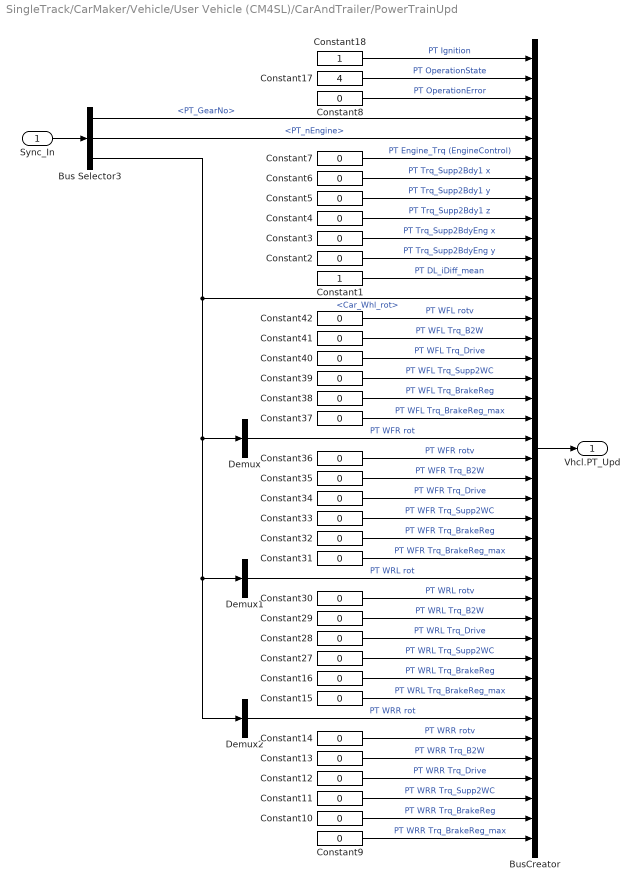
== system SingleTrack/CarMaker/Vehicle/User Vehicle (CM4SL)/CarAndTrailer/PowerTrainUpd ==
  Sync_In : Inport  OutDataType=sfix(16)  OutScaling=2^0
  Bus Selector3 : BusSelector  OutputSignals=PT_GearNo,PT_nEngine,Car_Whl_rot
  BusCreator : BusCreator  Inputs=40
  Constant1 : Constant  OutDataType=sfix(16)  OutScaling=2^0
  Constant{2..16,27..42} (31 alike) : Constant  Value=0  OutDataType=sfix(16)  OutScaling=2^0
  Constant17 : Constant  Value=4  OutDataType=sfix(16)  OutScaling=2^0
  Constant18 : Constant  OutDataType=sfix(16)  OutScaling=2^0
  Demux : Demux  Outputs=1
  Demux1 : Demux  Outputs=1
  Demux2 : Demux  Outputs=1
  Vhcl.PT_Upd : Outport  OutDataType=sfix(16)  OutScaling=2^0
  wires:
  Sync_In/1 -> Bus Selector3/1
  Bus Selector3/2 -> BusCreator/5  "<PT_nEngine>"
  Bus Selector3/1 -> BusCreator/4  "<PT_GearNo>"
  Bus Selector3/3 -> Demux/1, Demux1/1, Demux2/1, BusCreator/13  "<Car_Whl_rot>"
  Demux2/1 -> BusCreator/34  "PT WRR rot"
  Demux1/1 -> BusCreator/27  "PT WRL rot"
  Demux/1 -> BusCreator/20  "PT WFR rot"
  Constant9/1 -> BusCreator/40  "PT WRR Trq_BrakeReg_max"
  Constant10/1 -> BusCreator/39  "PT WRR Trq_BrakeReg"
  Constant11/1 -> BusCreator/38  "PT WRR Trq_Supp2WC"
  Constant12/1 -> BusCreator/37  "PT WRR Trq_Drive"
  Constant13/1 -> BusCreator/36  "PT WRR Trq_B2W"
  Constant14/1 -> BusCreator/35  "PT WRR rotv"
  Constant15/1 -> BusCreator/33  "PT WRL Trq_BrakeReg_max"
  Constant16/1 -> BusCreator/32  "PT WRL Trq_BrakeReg"
  Constant27/1 -> BusCreator/31  "PT WRL Trq_Supp2WC"
  Constant28/1 -> BusCreator/30  "PT WRL Trq_Drive"
  Constant29/1 -> BusCreator/29  "PT WRL Trq_B2W"
  Constant30/1 -> BusCreator/28  "PT WRL rotv"
  Constant31/1 -> BusCreator/26  "PT WFR Trq_BrakeReg_max"
  Constant32/1 -> BusCreator/25  "PT WFR Trq_BrakeReg"
  Constant33/1 -> BusCreator/24  "PT WFR Trq_Supp2WC"
  Constant34/1 -> BusCreator/23  "PT WFR Trq_Drive"
  Constant35/1 -> BusCreator/22  "PT WFR Trq_B2W"
  Constant36/1 -> BusCreator/21  "PT WFR rotv"
  Constant37/1 -> BusCreator/19  "PT WFL Trq_BrakeReg_max"
  Constant38/1 -> BusCreator/18  "PT WFL Trq_BrakeReg"
  Constant39/1 -> BusCreator/17  "PT WFL Trq_Supp2WC"
  Constant40/1 -> BusCreator/16  "PT WFL Trq_Drive"
  Constant41/1 -> BusCreator/15  "PT WFL Trq_B2W"
  Constant42/1 -> BusCreator/14  "PT WFL rotv"
  Constant1/1 -> BusCreator/12  "PT DL_iDiff_mean"
  Constant2/1 -> BusCreator/11  "PT Trq_Supp2BdyEng y"
  Constant3/1 -> BusCreator/10  "PT Trq_Supp2BdyEng x"
  Constant4/1 -> BusCreator/9  "PT Trq_Supp2Bdy1 z"
  Constant5/1 -> BusCreator/8  "PT Trq_Supp2Bdy1 y"
  Constant6/1 -> BusCreator/7  "PT Trq_Supp2Bdy1 x"
  Constant7/1 -> BusCreator/6  "PT Engine_Trq (EngineControl)"
  Constant8/1 -> BusCreator/3  "PT OperationError"
  Constant17/1 -> BusCreator/2  "PT OperationState"
  Constant18/1 -> BusCreator/1  "PT Ignition"
  BusCreator/1 -> Vhcl.PT_Upd/1

== system SingleTrack/CarMaker/Vehicle/User Vehicle (CM4SL)/CarAndTrailer/Query Road ==
  In1 : Inport  OutDataType=sfix(16)  OutScaling=2^0
  Bus Selector1 : BusSelector  OutputSignals=Car_Dist,Car_x,Car_y
  Bus Selector2 : BusSelector  OutputSignals=z,slope,grade,s
  Constant1 : Constant  Value=0  OutDataType=sfix(16)  OutScaling=2^0
  Constant2 : Constant  Value=0  OutDataType=sfix(16)  OutScaling=2^0
  IPGRoad5 : CarMaker4SL/IPGRoad5  SystemSampleTime=-1  xname=IPGRoad  xevalmode=RouteEval XY_S  xconsiderbumps=on  xusepath=off  xwithcurve=off  xabort=on
  Mux : Mux  Inputs=3
  Mux1 : Mux  Inputs=2
  Read CM Parameter : CarMaker4SL/Read CM Parameter  xfile=Vehicle  xkey=Wheel.fl.pos  xnout=1  xdefaults=0  xmuxed=on
  Sum2 : Sum  OutDataType=sfix(16)  OutScaling=2^0  SaturateOnIntegerOverflow=on  InputSameDT=on  OutDataTypeStr=Inherit: Same as first input
  Terminator : Terminator
  neg : Gain  Gain=-1  ParameterDataType=sfix(16)  ParameterScaling=2^0  OutDataType=sfix(16)  OutScaling=2^0  SaturateOnIntegerOverflow=on  OutDataTypeStr=Inherit: Same as input  ParamDataTypeStr=Inherit: Same as input
  Fr1_z : Outport  OutDataType=sfix(16)  OutScaling=2^0
  Fr1_rx : Outport  Port=2  OutDataType=sfix(16)  OutScaling=2^0
  Fr1_ry : Outport  Port=3  OutDataType=sfix(16)  OutScaling=2^0
  sRoad : Outport  Port=4  OutDataType=sfix(16)  OutScaling=2^0
  wires:
  Constant2/1 -> Mux/3
  Bus Selector2/2 -> Fr1_rx/1  "<slope>"
  Bus Selector2/1 -> Fr1_z/1  "<z>"
  In1/1 -> Bus Selector1/1
  Bus Selector1/1 -> Mux1/1  "<Car_Dist>"
  Mux/1 -> IPGRoad5/2
  Bus Selector1/3 -> Mux/2  "<Car_y>"
  Bus Selector1/2 -> Mux/1  "<Car_x>"
  IPGRoad5/2 -> Bus Selector2/1
  Constant1/1 -> Mux1/2
  Bus Selector2/3 -> neg/1  "<grade>"
  neg/1 -> Fr1_ry/1
  Bus Selector2/4 -> Sum2/1  "<s>"
  Sum2/1 -> sRoad/1
  Read CM Parameter/1 -> Sum2/2
  Mux1/1 -> IPGRoad5/1
  IPGRoad5/1 -> Terminator/1

== system SingleTrack/CarMaker/Vehicle/User Vehicle (CM4SL)/CarAndTrailer/SimStates ==
  note: Detect CarMaker states and transistions relevant for initialization at the start of a new testrun.
  Logical Operator : Logic  AllPortsSameDT=off  OutDataTypeMode=boolean  OutDataTypeStr=boolean
  Logical Operator1 : Logic  Operator=OR  AllPortsSameDT=off  OutDataTypeMode=boolean  OutDataTypeStr=boolean
  Memory : Memory
  Read CM Dict : CarMaker4SL/Read CM Dict  xname=SC.State  xsync=off
  Read CM Dict1 : CarMaker4SL/Read CM Dict  xname=Time  xsync=off
  Relational Operator : RelationalOperator  Operator=<=  LogicOutDataTypeMode=boolean  OutDataTypeStr=boolean
  Relational Operator1 : RelationalOperator  Operator===  LogicOutDataTypeMode=boolean  OutDataTypeStr=boolean
  Relational Operator2 : RelationalOperator  Operator===  LogicOutDataTypeMode=boolean  OutDataTypeStr=boolean
  SCState_Simulate : Constant  Value=8  OutDataType=sfix(16)  OutScaling=2^0
  Zero : Constant  Value=0  OutDataType=sfix(16)  OutScaling=2^0
  detect increase : RelationalOperator  Operator=>  LogicOutDataTypeMode=boolean  OutDataTypeStr=boolean
  tag scope: TRSim=global, TRStart=global
  wires:
  Read CM Dict/1 -> Relational Operator/1, Relational Operator1/2, Memory/1, detect increase/1
  SCState_Simulate/1 -> Relational Operator/2, Relational Operator1/1
  Relational Operator/1 -> Logical Operator/2
  Relational Operator1/1 -> [TRSim]
  Read CM Dict1/1 -> Relational Operator2/1
  Zero/1 -> Relational Operator2/2
  Relational Operator2/1 -> Logical Operator1/1
  Logical Operator/1 -> Logical Operator1/2
  Logical Operator1/1 -> [TRStart]
  detect increase/1 -> Logical Operator/1
  Memory/1 -> detect increase/2

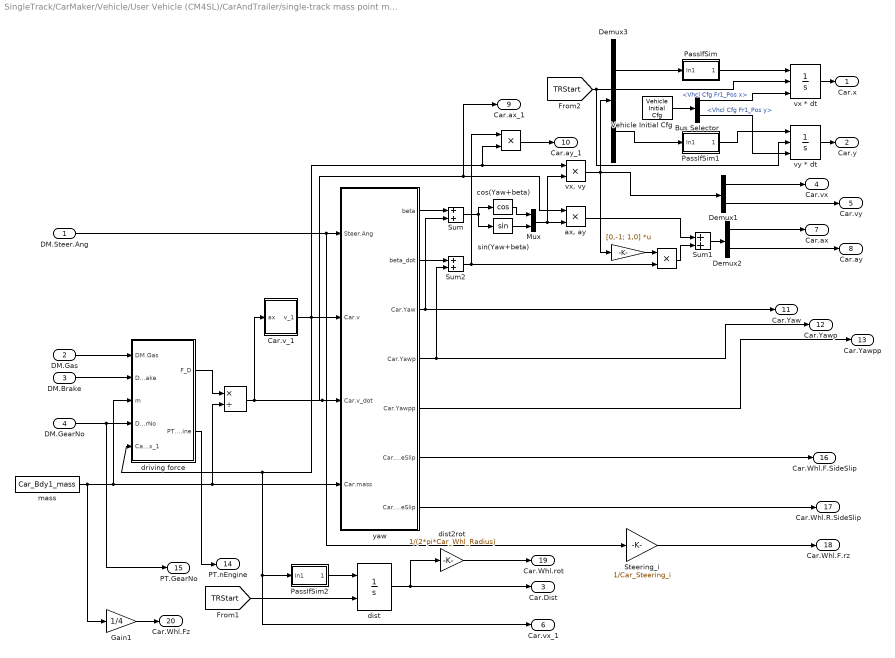
== system SingleTrack/CarMaker/Vehicle/User Vehicle (CM4SL)/CarAndTrailer/single-track mass point model ==
  DM.Steer.Ang : Inport  OutDataType=sfix(16)  OutScaling=2^0
  DM.Gas : Inport  Port=2  OutDataType=sfix(16)  OutScaling=2^0
  DM.Brake : Inport  Port=3  OutDataType=sfix(16)  OutScaling=2^0
  DM.GearNo : Inport  Port=4  OutDataType=sfix(16)  OutScaling=2^0
  " " : Gain  Gain=[0,-1; 1,0]  Multiplication=Matrix(K*u)  ParameterDataType=sfix(16)  ParameterScaling=2^0  OutDataType=sfix(16)  OutScaling=2^0  SaturateOnIntegerOverflow=on  OutDataTypeStr=Inherit: Same as input  ParamDataTypeStr=Inherit: Same as input
  "   " : Product  OutDataType=sfix(16)  OutScaling=2^0  SaturateOnIntegerOverflow=on  InputSameDT=on  OutDataTypeStr=Inherit: Same as first input
  "     " : Product  OutDataType=sfix(16)  OutScaling=2^0  SaturateOnIntegerOverflow=on  InputSameDT=on  OutDataTypeStr=Inherit: Same as first input
  "      " : Product  Inputs=*/  OutDataType=sfix(16)  OutScaling=2^0  SaturateOnIntegerOverflow=on  InputSameDT=on  OutDataTypeStr=Inherit: Same as first input
  Bus Selector : BusSelector  OutputSignals=Vhcl Cfg Fr1_Pos x,Vhcl Cfg Fr1_Pos y
  Car.v_1 : Subsystem
  Demux1 : Demux  Outputs=2
  Demux2 : Demux  Outputs=2
  Demux3 : Demux  Outputs=2
  Gain1 : Gain  Gain=1/4  ParameterDataType=sfix(16)  ParameterScaling=2^0  OutDataType=sfix(16)  OutScaling=2^0
  Mux : Mux  Inputs=2
  PassIfSim : Subsystem
  PassIfSim1 : Subsystem
  PassIfSim2 : Subsystem
  "Steering_i " : Gain  Gain=1/Car_Steering_i  ParameterDataType=sfix(16)  ParameterScaling=2^0  OutDataType=sfix(16)  OutScaling=2^0  SaturateOnIntegerOverflow=on  OutDataTypeStr=Inherit: Same as input  ParamDataTypeStr=Inherit: Same as input
  Sum : Sum  OutDataType=sfix(16)  OutScaling=2^0  SaturateOnIntegerOverflow=on  InputSameDT=on  OutDataTypeStr=Inherit: Same as first input
  Sum1 : Sum  OutDataType=sfix(16)  OutScaling=2^0  SaturateOnIntegerOverflow=on  InputSameDT=on  OutDataTypeStr=Inherit: Same as first input
  Sum2 : Sum  OutDataType=sfix(16)  OutScaling=2^0  SaturateOnIntegerOverflow=on  InputSameDT=on  OutDataTypeStr=Inherit: Same as first input
  Vehicle Initial Cfg : CarMaker4SL/Vehicle Initial Cfg  SystemSampleTime=-1
  "ax, ay" : Product  OutDataType=sfix(16)  OutScaling=2^0  SaturateOnIntegerOverflow=on  InputSameDT=on  OutDataTypeStr=Inherit: Same as first input
  cos(Yaw+beta) : Trigonometry  Operator=cos
  dist : Integrator  ExternalReset=level
  dist2rot : Gain  Gain=1/(2*pi*Car_Whl_Radius)  ParameterDataType=sfix(16)  ParameterScaling=2^0  OutDataType=sfix(16)  OutScaling=2^0  SaturateOnIntegerOverflow=on  OutDataTypeStr=Inherit: Same as input  ParamDataTypeStr=Inherit: Same as input
  driving force : Subsystem
  mass : Constant  Value=Car_Bdy1_mass  OutDataType=sfix(16)  OutScaling=2^0
  sin(Yaw+beta) : Trigonometry
  vx * dt : Integrator  ExternalReset=level  InitialConditionSource=external  InitialCondition=[0,0]
  "vx, vy" : Product  OutDataType=sfix(16)  OutScaling=2^0  SaturateOnIntegerOverflow=on  InputSameDT=on  OutDataTypeStr=Inherit: Same as first input
  vy * dt : Integrator  ExternalReset=level  InitialConditionSource=external  InitialCondition=[0,0]
  yaw : Subsystem
  Car.x : Outport  OutDataType=sfix(16)  OutScaling=2^0
  Car.y : Outport  Port=2  OutDataType=sfix(16)  OutScaling=2^0
  Car.Dist : Outport  Port=3  OutDataType=sfix(16)  OutScaling=2^0
  Car.vx : Outport  Port=4  OutDataType=sfix(16)  OutScaling=2^0
  Car.vy : Outport  Port=5  OutDataType=sfix(16)  OutScaling=2^0
  Car.vx_1 : Outport  Port=6  OutDataType=sfix(16)  OutScaling=2^0
  Car.ax : Outport  Port=7  OutDataType=sfix(16)  OutScaling=2^0
  Car.ay : Outport  Port=8  OutDataType=sfix(16)  OutScaling=2^0
  Car.ax_1 : Outport  Port=9  OutDataType=sfix(16)  OutScaling=2^0
  Car.ay_1 : Outport  Port=10  OutDataType=sfix(16)  OutScaling=2^0
  "Car.Yaw " : Outport  Port=11  OutDataType=sfix(16)  OutScaling=2^0
  Car.Yawp : Outport  Port=12  OutDataType=sfix(16)  OutScaling=2^0
  Car.Yawpp : Outport  Port=13  OutDataType=sfix(16)  OutScaling=2^0
  PT.nEngine : Outport  Port=14  OutDataType=sfix(16)  OutScaling=2^0
  PT.GearNo : Outport  Port=15  OutDataType=sfix(16)  OutScaling=2^0
  Car.Whl.F.SideSlip : Outport  Port=16  OutDataType=sfix(16)  OutScaling=2^0
  Car.Whl.R.SideSlip : Outport  Port=17  OutDataType=sfix(16)  OutScaling=2^0
  Car.Whl.F.rz : Outport  Port=18  OutDataType=sfix(16)  OutScaling=2^0
  Car.Whl.rot : Outport  Port=19  OutDataType=sfix(16)  OutScaling=2^0
  Car.Whl.Fz : Outport  Port=20  OutDataType=sfix(16)  OutScaling=2^0
  wires:
  [TRStart] -> dist/2
  PassIfSim2/1(Out1) -> dist/1
  PassIfSim1/1(Out1) -> vy * dt/1
  Demux3/2 -> PassIfSim1/1(In1)
  PassIfSim/1(Out1) -> vx * dt/1
  Demux3/1 -> PassIfSim/1(In1)
  dist2rot/1 -> Car.Whl.rot/1
  "Steering_i "/1 -> Car.Whl.F.rz/1
  driving force/2(PT.nEngine) -> PT.nEngine/1
  mass/1 -> "      "/2, yaw/4(Car.mass), driving force/3(m), Gain1/1
  DM.GearNo/1 -> PT.GearNo/1, driving force/4(DM.GearNo)
  Demux1/1 -> Car.vx/1
  dist/1 -> dist2rot/1, Car.Dist/1
  Demux2/2 -> Car.ay/1
  Demux2/1 -> Car.ax/1
  Demux1/2 -> Car.vy/1
  DM.Gas/1 -> driving force/1(DM.Gas)
  DM.Brake/1 -> driving force/2(DM.Brake)
  driving force/1(F_D) -> "      "/1
  "      "/1 -> "ax, ay"/1, Car.ax_1/1, yaw/3(Car.v_dot), Car.v_1/1(ax)
  yaw/7(Car.Whl.SideSlip) -> Car.Whl.R.SideSlip/1
  yaw/6(Car.Whl.F.SideSlip) -> Car.Whl.F.SideSlip/1
  DM.Steer.Ang/1 -> "Steering_i "/1, yaw/1(Steer.Ang)
  "     "/1 -> Car.ay_1/1
  " "/1 -> "   "/1
  Sum2/1 -> "     "/1, "   "/2
  yaw/2(beta_dot) -> Sum2/1
  "ax, ay"/1 -> Sum1/1
  "   "/1 -> Sum1/2
  Sum1/1 -> Demux2/1
  Car.v_1/1(v_1) -> PassIfSim2/1(In1), Car.vx_1/1, driving force/5(Car.vx_1), "     "/2, "vx, vy"/1, yaw/2(Car.v)
  "vx, vy"/1 -> " "/1, Demux1/1, Demux3/1
  Mux/1 -> "vx, vy"/2, "ax, ay"/2
  yaw/4(Car.Yawp) -> Sum2/2, Car.Yawp/1
  yaw/5(Car.Yawpp) -> Car.Yawpp/1
  Sum/1 -> sin(Yaw+beta)/1, cos(Yaw+beta)/1
  sin(Yaw+beta)/1 -> Mux/2
  cos(Yaw+beta)/1 -> Mux/1
  yaw/3(Car.Yaw) -> "Car.Yaw "/1, Sum/2
  yaw/1(beta) -> Sum/1
  [TRStart] -> vx * dt/2, vy * dt/2
  vy * dt/1 -> Car.y/1
  vx * dt/1 -> Car.x/1
  Vehicle Initial Cfg/1 -> Bus Selector/1
  Bus Selector/2 -> vy * dt/3  "<Vhcl Cfg Fr1_Pos y>"
  Bus Selector/1 -> vx * dt/3  "<Vhcl Cfg Fr1_Pos x>"
  Gain1/1 -> Car.Whl.Fz/1

== system SingleTrack/CarMaker/Vehicle/User Vehicle (ModelMgr)/Brake/CreateBus Vhcl.Wheel.PT ==
  In : Inport
  BusCreator : BusCreator  Inputs=16
  Demux : Demux  Outputs=16
  Out : Outport
  wires:
  In/1 -> Demux/1
  BusCreator/1 -> Out/1
  Demux/1 -> BusCreator/1  "Vhcl Wheel FL Trq_Brake"
  Demux/2 -> BusCreator/2  "Vhcl Wheel FL Trq_BrakeReg_trg"
  Demux/3 -> BusCreator/3  "Vhcl Wheel FL Trq_T2W"
  Demux/4 -> BusCreator/4  "Vhcl Wheel FL WhlBearing"
  Demux/5 -> BusCreator/5  "Vhcl Wheel FR Trq_Brake"
  Demux/6 -> BusCreator/6  "Vhcl Wheel FR Trq_BrakeReg_trg"
  Demux/7 -> BusCreator/7  "Vhcl Wheel FR Trq_T2W"
  Demux/8 -> BusCreator/8  "Vhcl Wheel FR WhlBearing"
  Demux/9 -> BusCreator/9  "Vhcl Wheel RL Trq_Brake"
  Demux/10 -> BusCreator/10  "Vhcl Wheel RL Trq_BrakeReg_trg"
  Demux/11 -> BusCreator/11  "Vhcl Wheel RL Trq_T2W"
  Demux/12 -> BusCreator/12  "Vhcl Wheel RL WhlBearing"
  Demux/13 -> BusCreator/13  "Vhcl Wheel RR Trq_Brake"
  Demux/14 -> BusCreator/14  "Vhcl Wheel RR Trq_BrakeReg_trg"
  Demux/15 -> BusCreator/15  "Vhcl Wheel RR Trq_T2W"
  Demux/16 -> BusCreator/16  "Vhcl Wheel RR WhlBearing"

== system SingleTrack/CarMaker/Vehicle/User Vehicle (ModelMgr)/CarAndTrailer/CarAndTrailerUpd ==
  Sync_In : Inport  OutDataType=sfix(16)  OutScaling=2^0
  Vhcl.Steering : Inport  Port=2  OutDataType=sfix(16)  OutScaling=2^0
  Vhcl.Motion : Inport  Port=3  OutDataType=sfix(16)  OutScaling=2^0
  Vhcl.PoI : Inport  Port=4  OutDataType=sfix(16)  OutScaling=2^0
  Vhcl.Wheel.FL : Inport  Port=5  OutDataType=sfix(16)  OutScaling=2^0
  Vhcl.Wheel.FR : Inport  Port=6  OutDataType=sfix(16)  OutScaling=2^0
  Vhcl.Wheel.RL : Inport  Port=7  OutDataType=sfix(16)  OutScaling=2^0
  Vhcl.Wheel.RR : Inport  Port=8  OutDataType=sfix(16)  OutScaling=2^0
  Car.Hitch.FrcTrq : Inport  Port=9  OutDataType=sfix(16)  OutScaling=2^0
  Vhcl.Fr1A : Inport  Port=10  OutDataType=sfix(16)  OutScaling=2^0
  CarAndTrailerUpd : S-Function  FunctionName=CM_Sfun  Parameters='CarAndTrUpd'  EnableBusSupport=off
  CreateBus Brake.IF.In : Subsystem
  Sync_Out : Outport  OutDataType=sfix(16)  OutScaling=2^0
  Brake.IF.In : Outport  Port=2  OutDataType=sfix(16)  OutScaling=2^0
  wires:
  Sync_In/1 -> CarAndTrailerUpd/1
  CarAndTrailerUpd/1 -> Sync_Out/1
  CreateBus Brake.IF.In/1(Out) -> Brake.IF.In/1
  CarAndTrailerUpd/2 -> CreateBus Brake.IF.In/1(In)
  Vhcl.Wheel.RL/1 -> CarAndTrailerUpd/7
  Vhcl.Wheel.RR/1 -> CarAndTrailerUpd/8
  Car.Hitch.FrcTrq/1 -> CarAndTrailerUpd/9
  Vhcl.Wheel.FR/1 -> CarAndTrailerUpd/6
  Vhcl.Wheel.FL/1 -> CarAndTrailerUpd/5
  Vhcl.PoI/1 -> CarAndTrailerUpd/4
  Vhcl.Motion/1 -> CarAndTrailerUpd/3
  Vhcl.Steering/1 -> CarAndTrailerUpd/2
  Vhcl.Fr1A/1 -> CarAndTrailerUpd/10  "user vehicle only"

== system SingleTrack/CarMaker/Vehicle/IPG Vehicle/CarAndTrailer/CarAndTrailerUpd/CreateBus Brake.IF.In ==
  In : Inport
  BusCreator : BusCreator  Inputs=9
  Demux : Demux  Outputs=9
  Out : Outport
  wires:
  In/1 -> Demux/1
  BusCreator/1 -> Out/1
  Demux/1 -> BusCreator/1  "Brake IF T_env"
  Demux/2 -> BusCreator/2  "Brake IF Trq_Reg_max FL"
  Demux/3 -> BusCreator/3  "Brake IF Trq_Reg_max FR"
  Demux/4 -> BusCreator/4  "Brake IF Trq_Reg_max RL"
  Demux/5 -> BusCreator/5  "Brake IF Trq_Reg_max RR"
  Demux/6 -> BusCreator/6  "Brake IF Trq_Reg FL"
  Demux/7 -> BusCreator/7  "Brake IF Trq_Reg FR"
  Demux/8 -> BusCreator/8  "Brake IF Trq_Reg RL"
  Demux/9 -> BusCreator/9  "Brake IF Trq_Reg RR"

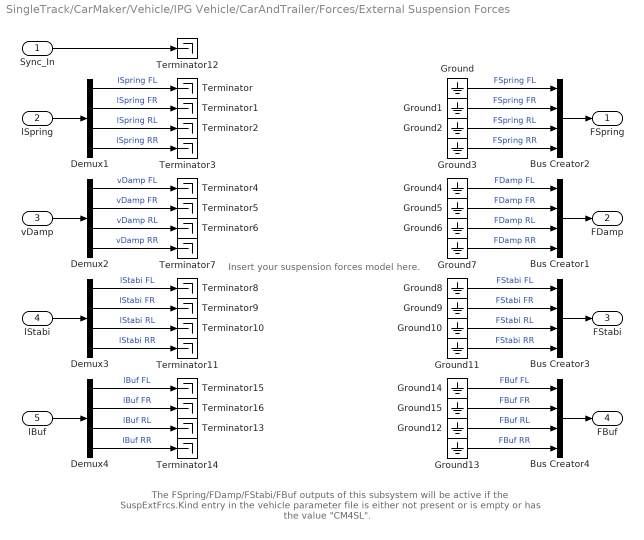
== system SingleTrack/CarMaker/Vehicle/IPG Vehicle/CarAndTrailer/Forces/External Suspension Forces ==
  note: Insert your suspension forces model here.
  note: The FSpring/FDamp/FStabi/FBuf outputs of this subsystem will be
      | active if the SuspExtFrcs.Kind entry in the vehicle parameter file
      | is either not present or is empty or has the value "CM4SL".
  Sync_In : Inport  OutDataType=sfix(16)  OutScaling=2^0
  lSpring : Inport  Port=2  OutDataType=sfix(16)  OutScaling=2^0
  vDamp : Inport  Port=3  OutDataType=sfix(16)  OutScaling=2^0
  lStabi : Inport  Port=4  OutDataType=sfix(16)  OutScaling=2^0
  lBuf : Inport  Port=5  OutDataType=sfix(16)  OutScaling=2^0
  Bus Creator{1..4} (4 alike) : BusCreator
  Demux{1..4} (4 alike) : Demux
  Ground{,1..15} (16 alike) : Ground
  Terminator{,1..16} (17 alike) : Terminator
  FSpring : Outport  OutDataType=sfix(16)  OutScaling=2^0
  FDamp : Outport  Port=2  OutDataType=sfix(16)  OutScaling=2^0
  FStabi : Outport  Port=3  OutDataType=sfix(16)  OutScaling=2^0
  FBuf : Outport  Port=4  OutDataType=sfix(16)  OutScaling=2^0
  wires:
  Bus Creator3/1 -> FStabi/1
  Ground11/1 -> Bus Creator3/4  "FStabi RR"
  Ground10/1 -> Bus Creator3/3  "FStabi RL"
  Ground9/1 -> Bus Creator3/2  "FStabi FR"
  Ground8/1 -> Bus Creator3/1  "FStabi FL"
  Bus Creator1/1 -> FDamp/1
  Ground7/1 -> Bus Creator1/4  "FDamp RR"
  Ground6/1 -> Bus Creator1/3  "FDamp RL"
  Ground5/1 -> Bus Creator1/2  "FDamp FR"
  Ground4/1 -> Bus Creator1/1  "FDamp FL"
  Ground3/1 -> Bus Creator2/4  "FSpring RR"
  Ground2/1 -> Bus Creator2/3  "FSpring RL"
  Ground1/1 -> Bus Creator2/2  "FSpring FR"
  Ground/1 -> Bus Creator2/1  "FSpring FL"
  Bus Creator2/1 -> FSpring/1
  Demux2/4 -> Terminator7/1  "vDamp RR"
  Demux2/3 -> Terminator6/1  "vDamp RL"
  Demux2/2 -> Terminator5/1  "vDamp FR"
  Demux2/1 -> Terminator4/1  "vDamp FL"
  Demux1/4 -> Terminator3/1  "lSpring RR"
  Demux1/3 -> Terminator2/1  "lSpring RL"
  Demux1/2 -> Terminator1/1  "lSpring FR"
  Demux1/1 -> Terminator/1  "lSpring FL"
  Demux3/4 -> Terminator11/1  "lStabi RR"
  Demux3/3 -> Terminator10/1  "lStabi RL"
  Demux3/2 -> Terminator9/1  "lStabi FR"
  Demux3/1 -> Terminator8/1  "lStabi FL"
  lStabi/1 -> Demux3/1
  vDamp/1 -> Demux2/1
  lSpring/1 -> Demux1/1
  Sync_In/1 -> Terminator12/1
  Bus Creator4/1 -> FBuf/1
  Ground13/1 -> Bus Creator4/4  "FBuf RR"
  Ground12/1 -> Bus Creator4/3  "FBuf RL"
  Ground15/1 -> Bus Creator4/2  "FBuf FR"
  Ground14/1 -> Bus Creator4/1  "FBuf FL"
  Demux4/4 -> Terminator14/1  "lBuf RR"
  Demux4/3 -> Terminator13/1  "lBuf RL"
  Demux4/2 -> Terminator16/1  "lBuf FR"
  Demux4/1 -> Terminator15/1  "lBuf FL"
  lBuf/1 -> Demux4/1
